simulink subsystem "s2s_to_3s"  (R2022b)
settings: Solver=VariableStepAuto  StartTime=0.0  StopTime=10.0  RelTol=1e-3
settings Model: Creator=jack  LastModifiedBy=jack

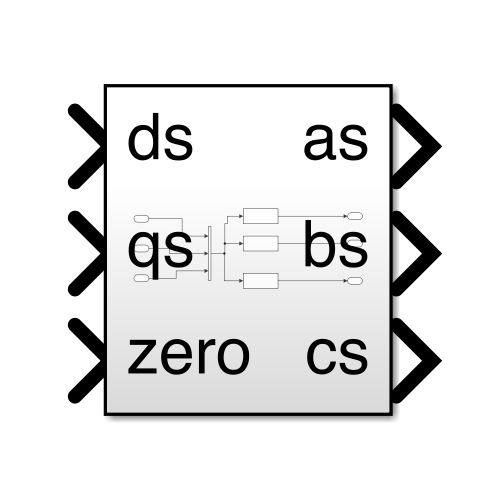
[thumbnail: Simulink's stored preview of the top-level diagram]
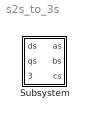
== system s2s_to_3s ==
  Subsystem : Subsystem

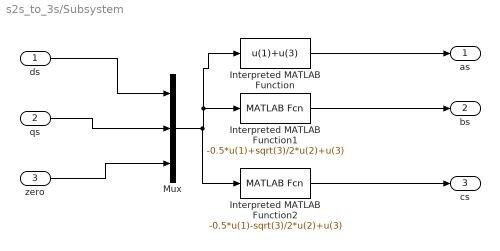
== system s2s_to_3s/Subsystem ==
  ds : Inport
  qs : Inport  Port=2
  zero : Inport  Port=3
  Interpreted MATLAB Function : MATLABFcn  MATLABFcn=u(1)+u(3)
  Interpreted MATLAB Function1 : MATLABFcn  MATLABFcn=-0.5*u(1)+sqrt(3)/2*u(2)+u(3)
  Interpreted MATLAB Function2 : MATLABFcn  MATLABFcn=-0.5*u(1)-sqrt(3)/2*u(2)+u(3)
  Mux : Mux  Inputs=3
  as : Outport
  bs : Outport  Port=2
  cs : Outport  Port=3
  wires:
  qs/1 -> Mux/2
  ds/1 -> Mux/1
  Mux/1 -> Interpreted MATLAB Function1/1, Interpreted MATLAB Function/1, Interpreted MATLAB Function2/1
  zero/1 -> Mux/3
  Interpreted MATLAB Function2/1 -> cs/1
  Interpreted MATLAB Function/1 -> as/1
  Interpreted MATLAB Function1/1 -> bs/1
